simulink model "Ch2_Simulink"  (R2024b)
settings: Solver=VariableStepAuto  StartTime=0.0  StopTime=10  RelTol=1e-3
values from neighbouring files (symbols this model uses):
  a_0_m_s2 = 1    [Ch2.m]
  v_0_m_s = 10    [Ch2.m]
  x_0_m = 5    [Ch2.m]
settings Model: Creator=veronicapranowo  LastModifiedBy=veronicapranowo

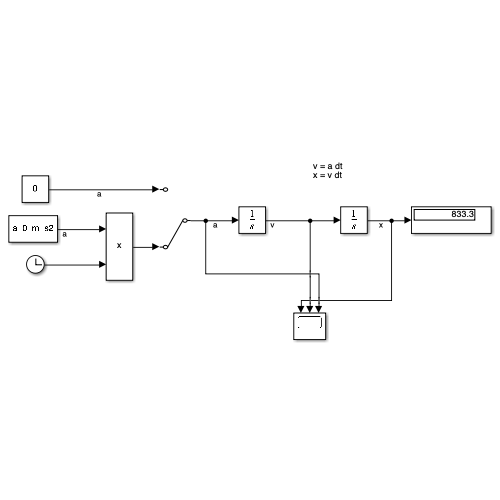
[thumbnail: Simulink's stored preview of the top-level diagram]
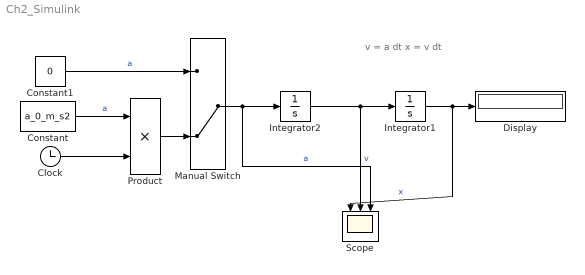
== system Ch2_Simulink ==
  note: v = a dt
      | x = v dt
  Clock : Clock
  Constant : Constant  Value=a_0_m_s2
  Constant1 : Constant  Value=0
  Display : Display
  Integrator1 : Integrator  InitialCondition=x_0_m
  Integrator2 : Integrator  InitialCondition=v_0_m_s
  Manual Switch : ManualSwitch  CurrentSetting=0
  Product : Product
  Scope : Scope  NumInputPorts=3
  wires:
  Integrator1/1 -> Scope/1, Display/1  "x"
  Integrator2/1 -> Scope/2, Integrator1/1  "v"
  Constant1/1 -> Manual Switch/1  "a"
  Manual Switch/1 -> Scope/3, Integrator2/1  "a"
  Clock/1 -> Product/2
  Constant/1 -> Product/1  "a"
  Product/1 -> Manual Switch/2
